simulink model "task1"  (Simulink 7.5)
settings: Solver=ode45  StartTime=0.0  StopTime=0.95  RelTol=1e-3
libraries: simulink x1
settings Model: Creator=Dranik_win  LastModifiedBy=Dranik_win

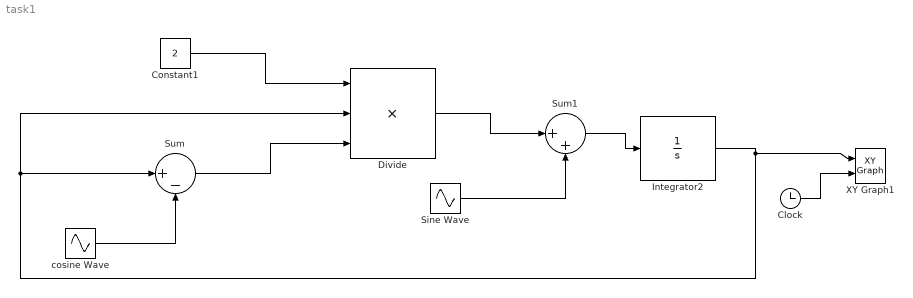
== system task1 ==
  Clock : Clock
      settings: Decimation=10
  Constant1 : Constant  Value=2  OutDataType=fixdt(1, 16)  OutScaling=2^0
  Divide : Product  Inputs=***  OutDataType=fixdt(1, 16)  OutScaling=2^-10
  Integrator2 : Integrator  InitialCondition=1
  Sine Wave : Sin  Amplitude=1  Bias=0  Frequency=1  Phase=0  Samples=10  SampleTime=0  Offset=0
  Sum : Sum  Inputs=|+-  OutDataType=fixdt(1, 16)  OutScaling=2^0
  Sum1 : Sum  Inputs=|++  OutDataType=fixdt(1, 16)  OutScaling=2^0
  XY Graph1 : simulink/Sinks/XY Graph  SystemSampleTime=-1  xmin=1  xmax=1.95  ymin=0  ymax=3  st=-1
  cosine Wave : Sin  Amplitude=1  Bias=0  Frequency=1  Phase=pi/2  Samples=10  SampleTime=0  Offset=0
  wires:
  Sum/1 -> Divide/3
  Constant1/1 -> Divide/1
  cosine Wave/1 -> Sum/2
  Divide/1 -> Sum1/1
  Sum1/1 -> Integrator2/1
  Integrator2/1 -> Sum/1, Divide/2, XY Graph1/1
  Clock/1 -> XY Graph1/2
  Sine Wave/1 -> Sum1/2
